simulink model "ArticulatedVehicleSimulink"  (R2015a)
settings: Solver=ode45  StartTime=0.0  StopTime=10.0  RelTol=1e-3
settings Model: Creator=andre  LastModifiedBy=root
settings DebuggingCC: UnderspecifiedInitializationDetection=Classic  MergeDetectMultiDrivingBlocksExec=none  SolverPrmCheckMsg=warning  StateNameClashWarn=warning

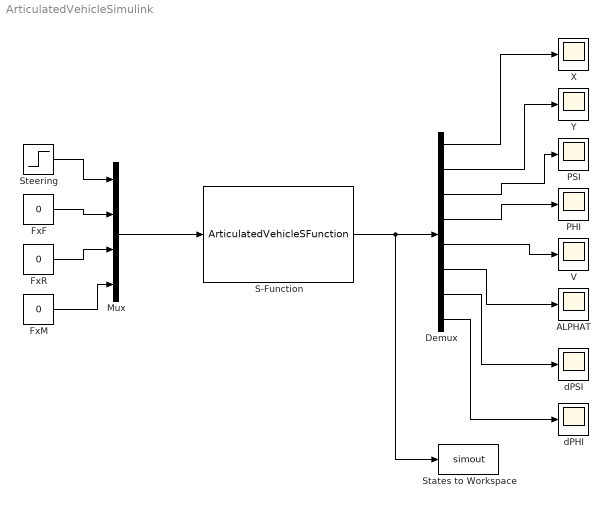
== system ArticulatedVehicleSimulink ==
  ALPHAT : Scope
      settings: SaveName=ScopeData5
  Demux : Demux  Outputs=8
  FxF : Constant  Value=0
  FxM : Constant  Value=0
  FxR : Constant  Value=0
  Mux : Mux
  PHI : Scope
      settings: SaveName=ScopeData3
  PSI : Scope
      settings: SaveName=ScopeData2
  S-Function : S-Function  FunctionName=ArticulatedVehicleSFunction
  States to Workspace : ToWorkspace  VariableName=simout  SaveFormat=Timeseries  SampleTime=-1
  Steering : Step  After=5*pi/180  SampleTime=0
  V : Scope
      settings: SaveName=ScopeData4
  X : Scope
  Y : Scope
  dPHI : Scope
      settings: SaveName=ScopeData7
  dPSI : Scope
      settings: SaveName=ScopeData6
  wires:
  Steering/1 -> Mux/1
  FxF/1 -> Mux/2
  FxR/1 -> Mux/3
  Mux/1 -> S-Function/1
  S-Function/1 -> States to Workspace/1, Demux/1
  Demux/1 -> X/1
  Demux/2 -> Y/1
  Demux/3 -> PSI/1
  Demux/4 -> PHI/1
  Demux/5 -> V/1
  Demux/6 -> ALPHAT/1
  FxM/1 -> Mux/4
  Demux/7 -> dPSI/1
  Demux/8 -> dPHI/1
